simulink model "symodel"  (R2017a)
settings: Solver=FixedStepAuto  StartTime=0.0  StopTime=stoptime  FixedStep=timestep  RelTol=1e-3
undefined symbols (not defined in the file): alpha, amplitude, fnoise, fseed, gain, omega0, phi0, prx, reff, snoise, sseed, tau, tau_match, tau_mzi, timestep
libraries: simulink x4
settings Model: Creator=taehwan  LastModifiedBy=taehwan

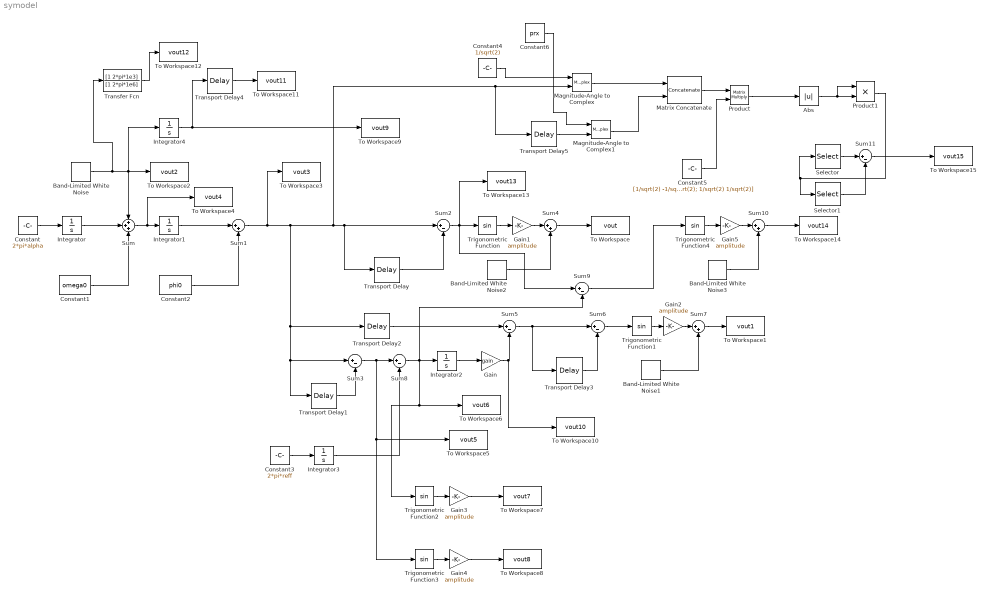
== system symodel ==
  Abs : Abs
  Band-Limited White Noise : simulink/Sources/Band-Limited White Noise  Cov=[fnoise*2*pi]  Ts=timestep  seed=[fseed]
  Band-Limited White Noise1 : simulink/Sources/Band-Limited White Noise  Cov=[snoise]  Ts=timestep  seed=[sseed]
  Band-Limited White Noise2 : simulink/Sources/Band-Limited White Noise  Cov=[snoise]  Ts=timestep  seed=[sseed]
  Band-Limited White Noise3 : simulink/Sources/Band-Limited White Noise  Cov=[snoise]  Ts=timestep  seed=[sseed]
  Constant : Constant  Value=2*pi*alpha
  Constant1 : Constant  Value=omega0
  Constant2 : Constant  Value=phi0
  Constant3 : Constant  Value=2*pi*reff
  Constant4 : Constant  Value=1/sqrt(2)
  Constant5 : Constant  Value=[1/sqrt(2) -1/sqrt(2); 1/sqrt(2) 1/sqrt(2)]
  Constant6 : Constant  Value=prx
  Gain : Gain  Gain=gain
  Gain{1..5} (5 alike) : Gain  Gain=amplitude
  Integrator{,1..4} (5 alike) : Integrator
  Magnitude-Angle to Complex : MagnitudeAngleToComplex
  Magnitude-Angle to Complex1 : MagnitudeAngleToComplex
  Matrix Concatenate : Concatenate  Mode=Multidimensional array  ConcatenateDimension=2
  Product : Product  Multiplication=Matrix(*)
  Product1 : Product
  Selector : Selector  InputPortWidth=2  IndexOptions=Index vector (dialog)  Indices=[1]  OutputSizes=1
  Selector1 : Selector  InputPortWidth=2  IndexOptions=Index vector (dialog)  Indices=[2]  OutputSizes=1
  Sum : Sum  Inputs=+++
  Sum{1,4,7,10} (4 alike) : Sum  Inputs=|++
  Sum{2..3,5..6,8..9,11} (7 alike) : Sum  Inputs=|+-
  To Workspace : ToWorkspace  VariableName=vout  SaveFormat=Timeseries  SampleTime=-1
  To Workspace1 : ToWorkspace  VariableName=vout1  SaveFormat=Timeseries  SampleTime=-1
  To Workspace10 : ToWorkspace  VariableName=vout10  SaveFormat=Timeseries  SampleTime=-1
  To Workspace11 : ToWorkspace  VariableName=vout11  SaveFormat=Timeseries  SampleTime=-1
  To Workspace12 : ToWorkspace  VariableName=vout12  SaveFormat=Timeseries  SampleTime=-1
  To Workspace13 : ToWorkspace  VariableName=vout13  SaveFormat=Timeseries  SampleTime=-1
  To Workspace14 : ToWorkspace  VariableName=vout14  SaveFormat=Timeseries  SampleTime=-1
  To Workspace15 : ToWorkspace  VariableName=vout15  SaveFormat=Timeseries  SampleTime=-1
  To Workspace2 : ToWorkspace  VariableName=vout2  SaveFormat=Timeseries  SampleTime=-1
  To Workspace3 : ToWorkspace  VariableName=vout3  SaveFormat=Timeseries  SampleTime=-1
  To Workspace4 : ToWorkspace  VariableName=vout4  SaveFormat=Timeseries  SampleTime=-1
  To Workspace5 : ToWorkspace  VariableName=vout5  SaveFormat=Timeseries  SampleTime=-1
  To Workspace6 : ToWorkspace  VariableName=vout6  SaveFormat=Timeseries  SampleTime=-1
  To Workspace7 : ToWorkspace  VariableName=vout7  SaveFormat=Timeseries  SampleTime=-1
  To Workspace8 : ToWorkspace  VariableName=vout8  SaveFormat=Timeseries  SampleTime=-1
  To Workspace9 : ToWorkspace  VariableName=vout9  SaveFormat=Timeseries  SampleTime=-1
  Transfer Fcn : TransferFcn  Numerator=[1 2*pi*1e3]  Denominator=[1 2*pi*1e6]
  Transport Delay : TransportDelay  DelayTime=tau  BufferSize=4096
  Transport Delay1 : TransportDelay  DelayTime=tau_mzi  BufferSize=4096
  Transport Delay2 : TransportDelay  DelayTime=tau_match  BufferSize=4096
  Transport Delay3 : TransportDelay  DelayTime=tau  BufferSize=4096
  Transport Delay4 : TransportDelay  DelayTime=tau_match  BufferSize=4096
  Transport Delay5 : TransportDelay  DelayTime=tau  BufferSize=4096
  Trigonometric Function{,1..4} (5 alike) : Trigonometry  OutputSignalType=real
  wires:
  Constant/1 -> Integrator/1
  Sum/1 -> To Workspace4/1, Integrator1/1
  Integrator1/1 -> Sum1/1
  Constant2/1 -> Sum1/2
  Transport Delay/1 -> Sum2/2
  Sum2/1 -> Sum9/1, To Workspace13/1, Trigonometric Function/1
  Sum1/1 -> To Workspace3/1, Transport Delay2/1, Sum3/1, Transport Delay1/1, Transport Delay5/1, Magnitude-Angle to Complex/2, Transport Delay/1, Sum2/1
  Constant1/1 -> Sum/3
  Integrator/1 -> Sum/2
  Band-Limited White Noise/1 -> Transfer Fcn/1, Sum/1, Integrator4/1, To Workspace2/1
  Band-Limited White Noise2/1 -> Sum4/2
  Transport Delay1/1 -> Sum3/2
  Transport Delay2/1 -> Sum5/1
  Sum5/1 -> Sum6/1, Transport Delay3/1
  Sum6/1 -> Trigonometric Function1/1
  Band-Limited White Noise1/1 -> Sum7/2
  Transport Delay3/1 -> Sum6/2
  Sum7/1 -> To Workspace1/1
  Sum8/1 -> Sum9/2, To Workspace6/1, Trigonometric Function2/1, Integrator2/1
  Constant3/1 -> Integrator3/1
  Integrator3/1 -> Sum8/2
  Integrator2/1 -> Gain/1
  Gain/1 -> To Workspace10/1, Sum5/2
  Sum4/1 -> To Workspace/1
  Trigonometric Function/1 -> Gain1/1
  Gain1/1 -> Sum4/1
  Trigonometric Function1/1 -> Gain2/1
  Gain2/1 -> Sum7/1
  Sum3/1 -> Trigonometric Function3/1, To Workspace5/1, Sum8/1
  Trigonometric Function2/1 -> Gain3/1
  Gain3/1 -> To Workspace7/1
  Trigonometric Function3/1 -> Gain4/1
  Gain4/1 -> To Workspace8/1
  Integrator4/1 -> Transport Delay4/1, To Workspace9/1
  Transport Delay4/1 -> To Workspace11/1
  Transfer Fcn/1 -> To Workspace12/1
  Sum10/1 -> To Workspace14/1
  Trigonometric Function4/1 -> Gain5/1
  Gain5/1 -> Sum10/1
  Band-Limited White Noise3/1 -> Sum10/2
  Sum9/1 -> Trigonometric Function4/1
  Magnitude-Angle to Complex/1 -> Matrix Concatenate/1
  Constant4/1 -> Magnitude-Angle to Complex/1
  Constant5/1 -> Product/2
  Transport Delay5/1 -> Magnitude-Angle to Complex1/2
  Matrix Concatenate/1 -> Product/1
  Product/1 -> Abs/1
  Selector/1 -> Sum11/1
  Selector1/1 -> Sum11/2
  Sum11/1 -> To Workspace15/1
  Constant6/1 -> Magnitude-Angle to Complex1/1
  Magnitude-Angle to Complex1/1 -> Matrix Concatenate/2
  Abs/1 -> Product1/2, Product1/1
  Product1/1 -> Selector1/1, Selector/1
